simulink model "TWFL_V1"  (R2025b)
settings: Solver=daessc  StartTime=0.0  StopTime=20  RelTol=1e-3
undefined symbols (not defined in the file): dspblkCoreblockFVToolHelper, g, g_fork, g_lift, gcbh, Kd_fork, Kd_lift, Kp_fork, Kp_lift, lx, ly, lz, M, m_w, Mn_33, Mn_44, N, r, T_control, X, Y, Z
libraries: sm_lib x80, nesl_utility x21, simulink x5, slpidlib x1
(part 3 of 3)

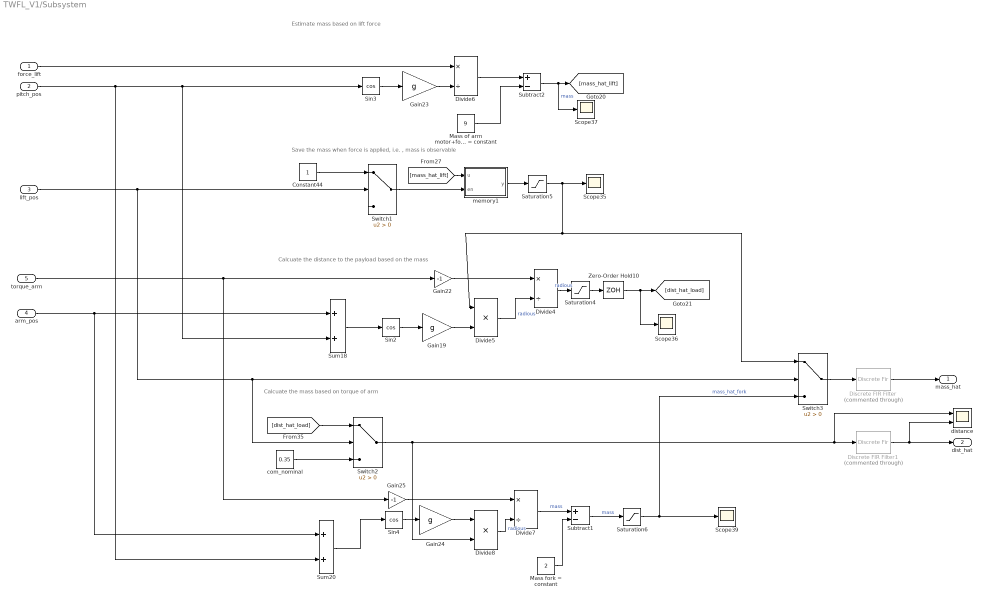
== system TWFL_V1/Subsystem ==
  note: Estimate mass based on lift force
  note: Save the mass when force is applied, i.e. , mass is observable
  note: Calcuate the distance to the payload based on the mass
  note: Calcuate the mass based on torque of arm
  force_lift : Inport
  pitch_pos : Inport  Port=2
  lift_pos : Inport  Port=3
  arm_pos : Inport  Port=4
  torque_arm : Inport  Port=5
  Constant44 : Constant
  Discrete FIR Filter : DiscreteFir  Commented=through  LoadFcn=dspblkCoreblockFVToolHelper(gcbh,'load');  Coefficients=ones(1,5000)/5000
      settings: CopyFcn=dspblkCoreblockFVToolHelper(gcbh,'copy');  DeleteFcn=dspblkCoreblockFVToolHelper(gcbh,'close');  ModelCloseFcn=dspblkCoreblockFVToolHelper(gcbh,'close');  PreSaveFcn=dspblkCoreblockFVToolHelper(gcbh,'presave');  PostSaveFcn=dspblkCoreblockFVToolHelper(gcbh,'postsave');  CloseFcn=dspblkCoreblockFVToolHelper(gcbh,'close');
  Discrete FIR Filter1 : DiscreteFir  Commented=through  LoadFcn=dspblkCoreblockFVToolHelper(gcbh,'load');  Coefficients=ones(1,500)/500
      settings: CopyFcn=dspblkCoreblockFVToolHelper(gcbh,'copy');  DeleteFcn=dspblkCoreblockFVToolHelper(gcbh,'close');  ModelCloseFcn=dspblkCoreblockFVToolHelper(gcbh,'close');  PreSaveFcn=dspblkCoreblockFVToolHelper(gcbh,'presave');  PostSaveFcn=dspblkCoreblockFVToolHelper(gcbh,'postsave');  CloseFcn=dspblkCoreblockFVToolHelper(gcbh,'close');
  Divide4 : Product  Inputs=*/
  Divide5 : Product  Inputs=**
  Divide6 : Product  Inputs=*/
  Divide7 : Product  Inputs=*/
  Divide8 : Product  Inputs=**
  Gain19 : Gain  Gain=g
  Gain22 : Gain  Gain=-1
  Gain23 : Gain  Gain=g
  Gain24 : Gain  Gain=g
  Gain25 : Gain  Gain=-1
  Mass fork = constant : Constant  Value=2
  Mass of arm motor+fork = constant : Constant  Value=9
  Saturation4 : Saturate  UpperLimit=0.6  LowerLimit=0.1
  Saturation5 : Saturate  UpperLimit=20  LowerLimit=0.001
  Saturation6 : Saturate  UpperLimit=20  LowerLimit=0
  Scope{35..37,39} (4 alike) : Scope
      Scope35 settings: ActiveDisplayYMinimum=-1.2708762754885328  ActiveDisplayYMaximum=14.804410070172921  DataLoggingVariableName=ScopeData41
      Scope36 settings: ActiveDisplayYMinimum=-0.0615737983063222  ActiveDisplayYMaximum=3.0231286948708305  DataLoggingVariableName=ScopeData42
      Scope37 settings: ActiveDisplayYMinimum=-4.9295636501203735  ActiveDisplayYMaximum=16.727099942606021  DataLoggingVariableName=ScopeData43
      Scope39 settings: ActiveDisplayYMinimum=-0.718038981848304  ActiveDisplayYMaximum=31.278716537533729  DataLoggingVariableName=ScopeData45
  Sin2 : Trigonometry  Operator=cos
  Sin3 : Trigonometry  Operator=cos
  Sin4 : Trigonometry  Operator=cos
  Subtract1 : Sum  Inputs=+-
  Subtract2 : Sum  Inputs=+-
  Sum18 : Sum
  Sum20 : Sum
  Switch1 : Switch  Criteria=u2 > Threshold  SaturateOnIntegerOverflow=off  InputSameDT=off
  Switch2 : Switch  Criteria=u2 > Threshold  SaturateOnIntegerOverflow=off  InputSameDT=off
  Switch3 : Switch  Criteria=u2 > Threshold  SaturateOnIntegerOverflow=off  InputSameDT=off
  Zero-Order Hold10 : ZeroOrderHold  SampleTime=-1
  com_nominal : Constant  Value=0.35
  distance : Scope  NumInputPorts=2
      settings: ActiveDisplayYMinimum=0.1935434288070958  ActiveDisplayYMaximum=0.90699580975947647  DataLoggingVariableName=ScopeData47
  memory1 : MATLAB Function  TreatAsAtomicUnit=on
  mass_hat : Outport
  dist_hat : Outport  Port=2
  wires:
  Constant44/1 -> Switch1/1
  memory1/1(y) -> Saturation5/1
  pitch_pos/1 -> Sum20/2, Sin3/1, Sum18/2
  lift_pos/1 -> Switch1/2, Switch2/2, Switch3/2
  com_nominal/1 -> Switch2/3
  Divide5/1 -> Divide4/2  "radious"
  force_lift/1 -> Divide6/1
  [mass_hat_lift] -> memory1/1(u)
  Switch1/1 -> memory1/2(en)
  Zero-Order Hold10/1 -> [dist_hat_load], Scope36/1
  [dist_hat_load] -> Switch2/1
  Sin4/1 -> Gain24/1
  Switch2/1 -> Discrete FIR Filter1/1, distance/1, Divide8/2
  Sin3/1 -> Gain23/1
  arm_pos/1 -> Sum20/1, Sum18/1
  Saturation5/1 -> Divide5/1, Switch3/1, Scope35/1
  Saturation4/1 -> Zero-Order Hold10/1
  Divide4/1 -> Saturation4/1  "radious"
  torque_arm/1 -> Gain22/1, Gain25/1
  Sum20/1 -> Sin4/1
  Saturation6/1 -> Switch3/3, Scope39/1  "mass_hat_fork"
  Sin2/1 -> Gain19/1
  Switch3/1 -> Discrete FIR Filter/1
  Gain25/1 -> Divide7/1
  Divide6/1 -> Subtract2/1
  Gain22/1 -> Divide4/1
  Divide7/1 -> Subtract1/1  "mass"
  Gain24/1 -> Divide8/1
  Divide8/1 -> Divide7/2  "radious"
  Mass of arm motor+fork = constant/1 -> Subtract2/2
  Sum18/1 -> Sin2/1
  Gain19/1 -> Divide5/2
  Subtract2/1 -> Scope37/1, [mass_hat_lift]  "mass"
  Gain23/1 -> Divide6/2
  Mass fork = constant/1 -> Subtract1/2
  Subtract1/1 -> Saturation6/1  "mass"
  Discrete FIR Filter1/1 -> distance/2, dist_hat/1
  Discrete FIR Filter/1 -> mass_hat/1

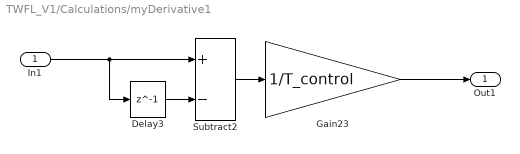
== system TWFL_V1/Calculations/myDerivative1 ==
  In1 : Inport
  Delay3 : Delay  DelayLength=1  InputProcessing=Columns as channels (frame based)
  Gain23 : Gain  Gain=1/T_control
  Subtract2 : Sum  Inputs=+-
  Out1 : Outport
  wires:
  Gain23/1 -> Out1/1
  Subtract2/1 -> Gain23/1
  Delay3/1 -> Subtract2/2
  In1/1 -> Subtract2/1, Delay3/1

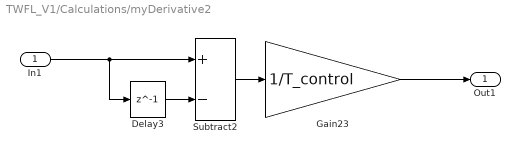
== system TWFL_V1/Calculations/myDerivative2 ==
  In1 : Inport
  Delay3 : Delay  DelayLength=1  InputProcessing=Columns as channels (frame based)
  Gain23 : Gain  Gain=1/T_control
  Subtract2 : Sum  Inputs=+-
  Out1 : Outport
  wires:
  Gain23/1 -> Out1/1
  Subtract2/1 -> Gain23/1
  Delay3/1 -> Subtract2/2
  In1/1 -> Subtract2/1, Delay3/1

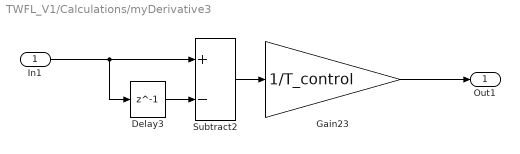
== system TWFL_V1/Calculations/myDerivative3 ==
  In1 : Inport
  Delay3 : Delay  DelayLength=1  InputProcessing=Columns as channels (frame based)
  Gain23 : Gain  Gain=1/T_control
  Subtract2 : Sum  Inputs=+-
  Out1 : Outport
  wires:
  In1/1 -> Delay3/1, Subtract2/1
  Delay3/1 -> Subtract2/2
  Subtract2/1 -> Gain23/1
  Gain23/1 -> Out1/1

== system TWFL_V1/Calculations/myDerivative4 ==
  In1 : Inport
  Delay3 : Delay  DelayLength=1  InputProcessing=Columns as channels (frame based)
  Gain23 : Gain  Gain=1/T_control
  Subtract2 : Sum  Inputs=+-
  Out1 : Outport
  wires:
  Gain23/1 -> Out1/1
  Subtract2/1 -> Gain23/1
  Delay3/1 -> Subtract2/2
  In1/1 -> Subtract2/1, Delay3/1

== system TWFL_V1/Calculations/myDerivative5 ==
  In1 : Inport
  Delay3 : Delay  DelayLength=1  InputProcessing=Columns as channels (frame based)
  Gain23 : Gain  Gain=1/T_control
  Subtract2 : Sum  Inputs=+-
  Out1 : Outport
  wires:
  In1/1 -> Delay3/1, Subtract2/1
  Delay3/1 -> Subtract2/2
  Subtract2/1 -> Gain23/1
  Gain23/1 -> Out1/1

== matlab function TWFL_V1/Subsystem/memory1 ==
  settings: updateMethod=DISCRETE
  data: u input; y output; en input
function y = fcn(u,en)
persistent mem
if isempty(mem)
    mem = 0; % valor inicial
end
if en
    mem = u;
end
y = mem;
end

== matlab function TWFL_V1/MATLAB Function1 ==
  settings: updateMethod=DISCRETE  sampleTime=T_control
  data: m_hat input; cdg output; pos_lift input; d_hat input; I_total output
function [cdg, I_total] = new_cdg_and_inertia(m_hat, pos_lift, d_hat)
%#codegen
% Compute total center of gravity and equivalent inertia (Y axis)
% Suitable for Simulink / code generation

% -------------------------------
% Fixed model parameters
% -------------------------------
m = [16.0;
     5.0;
     5.0;
     2.0;
     m_hat];

x = [ 0.0;
     -0.15;
     -0.10;
      0.30;
     -0.10 + d_hat];

z = [0.50;
     1.20 + pos_lift;
     1.05 + pos_lift;
     1.05 + pos_lift;
     1.05 + pos_lift];

I_y = [1.4533;
       0.9417;
       0.1531;
       0.0300;
       0.0000];

% -------------------------------
% Total mass
% -------------------------------
M = m(1) + m(2) + m(3) + m(4) + m(5);

% -------------------------------
% Center of gravity
% -------------------------------
x_G = (m(1)*x(1) + m(2)*x(2) + m(3)*x(3) + m(4)*x(4) + m(5)*x(5)) / M;
z_G = (m(1)*z(1) + m(2)*z(2) + m(3)*z(3) + m(4)*z(4) + m(5)*z(5)) / M;

cdg = [x_G; z_G];   % 2x1 vector (Simulink-friendly)

% -------------------------------
% Steiner inertia
% -------------------------------
dx1 = x(1) - x_G; dz1 = z(1) - z_G;
dx2 = x(2) - x_G; dz2 = z(2) - z_G;
dx3 = x(3) - x_G; dz3 = z(3) - z_G;
dx4 = x(4) - x_G; dz4 = z(4) - z_G;
dx5 = x(5) - x_G; dz5 = z(5) - z_G;

I_total = ...
    I_y(1) + m(1)*(dx1*dx1 + dz1*dz1) + ...
    I_y(2) + m(2)*(dx2*dx2 + dz2*dz2) + ...
    I_y(3) + m(3)*(dx3*dx3 + dz3*dz3) + ...
    I_y(4) + m(4)*(dx4*dx4 + dz4*dz4) + ...
    I_y(5) + m(5)*(dx5*dx5 + dz5*dz5);

end
